simulink model "FullModelSimulation"  (R2021b)
settings: Solver=VariableStepAuto  StartTime=0.0  StopTime=24*3600  RelTol=1e-3
values from neighbouring files (symbols this model uses):
  A = double(A)    [ComponentUnitTests.m]    (also in ComponentUnitTests_linerization.m; InnerLoopNonLinSim.m; Kalman_filter_v2.m = [-0.3236   -0.0406   -0.1577   10.0671   -0.7623    0.0000)
  K = 5.4274    [Kalman_filter_final.m]
  ts = 0.025    [ComponentUnitTests.m]    (also in ComponentUnitTests_linerization.m; InnerLoopNonLinSim.m; Kalman_filter_final.m = 1; Kalman_filter_v2.m)
undefined symbols (not defined in the file or in its folder): Bp, Discrete, Time
libraries: slpidlib x2, ctrlSharedLib x1, TankPressure_Lib x1, VelocityDALQR_lib x1
settings Model: Creator=Christian  LastModifiedBy=Christian
settings SolverCC: AlgebraicLoopSolver=TrustRegion
settings DebuggingCC: SFMachineParentedDataDiag=warning

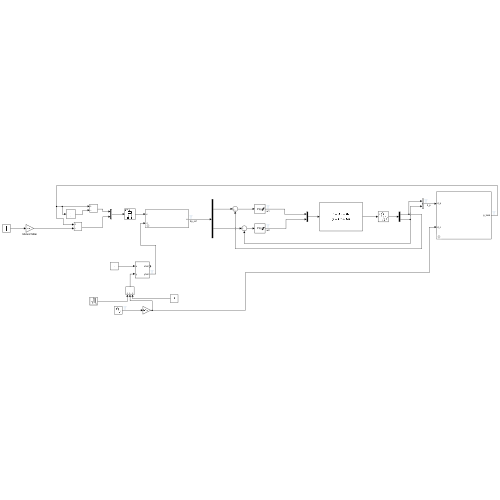
[thumbnail: Simulink's stored preview of the top-level diagram]
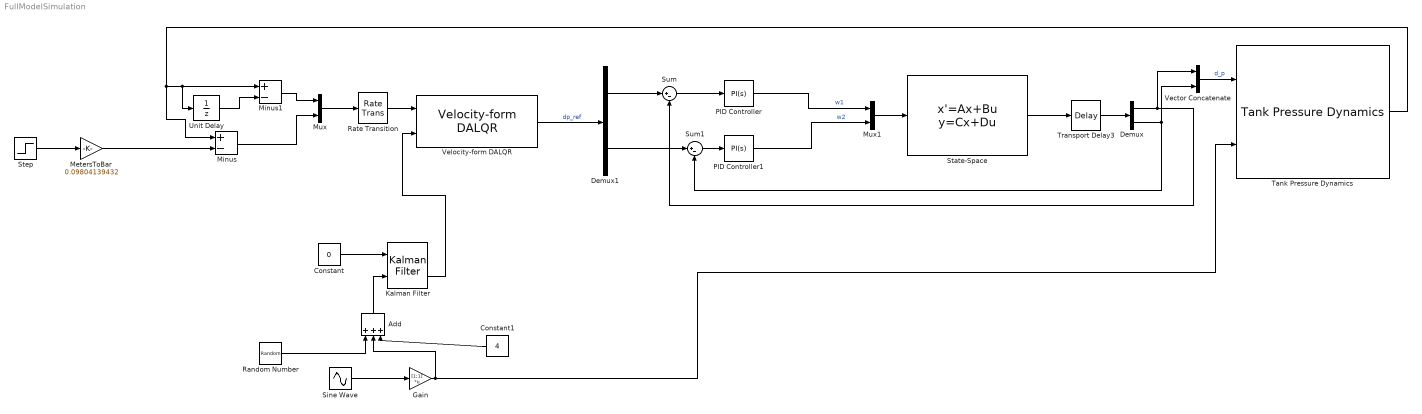
== system FullModelSimulation ==
  Add : Sum  Inputs=+++
  Constant : Constant  Value=0
  Constant1 : Constant  Value=4
  Demux : Demux  Outputs=2
  Demux1 : Demux  Outputs=2
  Gain : Gain  Gain=[1;1]  Multiplication=Matrix(K*u)
  Kalman Filter : ctrlSharedLib/Kalman Filter  TimeDomain=Discrete-Time  UseCurrentEstimator=on  ModelSource=LTI State-Space Variable  ModelSourceVariable=KalmSys  A=0.95  B=1  C=1  D=0  NumberOfStates=1  NumberOfInputs=1  NumberOfOutputs=1  InitialEstimateSource=Dialog  X0=0  P0=10  UseK=off  UseGH=off  NumberOfProcessNoiseInputs=1  G=1  TimeInvariantG=on  H=0  TimeInvariantH=on  Q=0.05  TimeInvariantQ=on  R=100  TimeInvariantR=on  N=0  TimeInvariantN=on  AddInputPort=on  AddEnablePort=off  OutputEstimatedY=on  OutputP=off  Ts=-1
  MetersToBar : Gain  Gain=0.09804139432
  Minus : Sum  Inputs=+-
  Minus1 : Sum  Inputs=+-
  Mux : Mux  Inputs=2
  Mux1 : Mux  Inputs=2
  PID Controller : slpidlib/PID Controller  Controller=PI  Form=Ideal  TimeDomain=Continuous-time  UseExternalTs=off  SampleTime=-1  IntegratorMethod=Forward Euler  FilterMethod=Forward Euler  ControllerParametersSource=internal  P=1.8  I=0.125  D=0  UseFilter=on  N=100  TunerSelectOption=Transfer Function Based (PID Tuner App)  InitialConditionSource=internal  InitialConditionForIntegrator=0  InitialConditionForFilter=0  DifferentiatorICPrevScaledInput=0  ExternalReset=none  TrackingMode=off  Kt=1  LimitOutput=on  SatLimitsSource=internal  UpperSaturationLimit=100  LowerSaturationLimit=0  LinearizeAsGain=on  AntiWindupMode=back-calculation  Kb=1  POutMin=[]  POutMax=[]  IOutMin=[]  IOutMax=[]  DOutMin=[]  DOutMax=[]  NOutMin=[]  NOutMax=[]  SumOutMin=[]  SumOutMax=[]  SaturationOutMin=[]  SaturationOutMax=[]  PParamMin=[]  PParamMax=[]  IParamMin=[]  IParamMax=[]  DParamMin=[]  DParamMax=[]  NParamMin=[]  NParamMax=[]  KbParamMin=[]  KbParamMax=[]  KtParamMin=[]  KtParamMax=[]  KbOutMin=[]  KbOutMax=[]  KtOutMin=[]  KtOutMax=[]  IntegratorOutMin=[]  IntegratorOutMax=[]  FilterOutMin=[]  FilterOutMax=[]  SumI1OutMin=[]  SumI1OutMax=[]  SumI2OutMin=[]  SumI2OutMax=[]  SumI3OutMin=[]  SumI3OutMax=[]  SumI4OutMin=[]  SumI4OutMax=[]  SumDOutMin=[]  SumDOutMax=[]  DifferentiatorOutMin=[]  DifferentiatorOutMax=[]  FilterDiffOutCoefMin=[]  FilterDiffOutCoefMax=[]  ReciprocalOutMin=[]  ReciprocalOutMax=[]  SumDenOutMin=[]  SumDenOutMax=[]  SumNumOutMin=[]  SumNumOutMax=[]  DivideOutMin=[]  DivideOutMax=[]  UdiffTsProdOutMin=[]  UdiffTsProdOutMax=[]  NTsProdOutMin=[]  NTsProdOutMax=[]  UintegralTsProdOutMin=[]  UintegralTsProdOutMax=[]  UngainTsProdOutMin=[]  UngainTsProdOutMax=[]  IntegratorContinuousStateAttributes=''  IntegratorStateMustResolveToSignalObject=off  IntegratorRTWStateStorageClass=Auto  FilterContinuousStateAttributes=''  FilterStateMustResolveToSignalObject=off  FilterRTWStateStorageClass=Auto  ParallelPVariant=Passthrough  IdealPVariant=InternalParameters  IVariant=InternalParameters  DVariant=Disabled  IntegratorVariant=Continuous  SatVariant=Enabled  AWVariant=BackCalculation  PCopyVariant=Disabled  TRVariant=Disabled  FdbkBlocksVariant=Forward  IdealPFdbkVariant=Disabled  SatFdbkVariant=Disabled  DerivativeFilterVariant=Disabled  NVariant=Disabled  NCopyVariant=Disabled_SignalSpec  FilterICVariant=Disabled  IntegratorICVariant=InternalICs  ExternalResetVariant=Disabled  TRSumVariant=Passthrough  SumFdbkVariant=Disabled  SumVariant=Sum_PI  TsampFilterVariant=InternalTs  TsampNgainVariant=Passthrough  TsampIntegralVariant=Passthrough  ExternalSaturationOutDataTypeStr=Inherit: Same as second input
  PID Controller1 : slpidlib/PID Controller  Controller=PI  Form=Ideal  TimeDomain=Continuous-time  UseExternalTs=off  SampleTime=-1  IntegratorMethod=Forward Euler  FilterMethod=Forward Euler  ControllerParametersSource=internal  P=1.8  I=0.125  D=0  UseFilter=on  N=100  TunerSelectOption=Transfer Function Based (PID Tuner App)  InitialConditionSource=internal  InitialConditionForIntegrator=0  InitialConditionForFilter=0  DifferentiatorICPrevScaledInput=0  ExternalReset=none  TrackingMode=off  Kt=1  LimitOutput=on  SatLimitsSource=internal  UpperSaturationLimit=100  LowerSaturationLimit=0  LinearizeAsGain=on  AntiWindupMode=back-calculation  Kb=1  POutMin=[]  POutMax=[]  IOutMin=[]  IOutMax=[]  DOutMin=[]  DOutMax=[]  NOutMin=[]  NOutMax=[]  SumOutMin=[]  SumOutMax=[]  SaturationOutMin=[]  SaturationOutMax=[]  PParamMin=[]  PParamMax=[]  IParamMin=[]  IParamMax=[]  DParamMin=[]  DParamMax=[]  NParamMin=[]  NParamMax=[]  KbParamMin=[]  KbParamMax=[]  KtParamMin=[]  KtParamMax=[]  KbOutMin=[]  KbOutMax=[]  KtOutMin=[]  KtOutMax=[]  IntegratorOutMin=[]  IntegratorOutMax=[]  FilterOutMin=[]  FilterOutMax=[]  SumI1OutMin=[]  SumI1OutMax=[]  SumI2OutMin=[]  SumI2OutMax=[]  SumI3OutMin=[]  SumI3OutMax=[]  SumI4OutMin=[]  SumI4OutMax=[]  SumDOutMin=[]  SumDOutMax=[]  DifferentiatorOutMin=[]  DifferentiatorOutMax=[]  FilterDiffOutCoefMin=[]  FilterDiffOutCoefMax=[]  ReciprocalOutMin=[]  ReciprocalOutMax=[]  SumDenOutMin=[]  SumDenOutMax=[]  SumNumOutMin=[]  SumNumOutMax=[]  DivideOutMin=[]  DivideOutMax=[]  UdiffTsProdOutMin=[]  UdiffTsProdOutMax=[]  NTsProdOutMin=[]  NTsProdOutMax=[]  UintegralTsProdOutMin=[]  UintegralTsProdOutMax=[]  UngainTsProdOutMin=[]  UngainTsProdOutMax=[]  IntegratorContinuousStateAttributes=''  IntegratorStateMustResolveToSignalObject=off  IntegratorRTWStateStorageClass=Auto  FilterContinuousStateAttributes=''  FilterStateMustResolveToSignalObject=off  FilterRTWStateStorageClass=Auto  ParallelPVariant=Passthrough  IdealPVariant=InternalParameters  IVariant=InternalParameters  DVariant=Disabled  IntegratorVariant=Continuous  SatVariant=Enabled  AWVariant=BackCalculation  PCopyVariant=Disabled  TRVariant=Disabled  FdbkBlocksVariant=Forward  IdealPFdbkVariant=Disabled  SatFdbkVariant=Disabled  DerivativeFilterVariant=Disabled  NVariant=Disabled  NCopyVariant=Disabled_SignalSpec  FilterICVariant=Disabled  IntegratorICVariant=InternalICs  ExternalResetVariant=Disabled  TRSumVariant=Passthrough  SumFdbkVariant=Disabled  SumVariant=Sum_PI  TsampFilterVariant=InternalTs  TsampNgainVariant=Passthrough  TsampIntegralVariant=Passthrough  ExternalSaturationOutDataTypeStr=Inherit: Same as second input
  Random Number : RandomNumber  Mean=[0;0]  Variance=[0.1;0.1]  SampleTime=10  VectorParams1D=off
  Rate Transition : RateTransition  OutPortSampleTime=100
  Sine Wave : Sin  Amplitude=2  Bias=-2  Frequency=2*pi*1/(12*3600)  SampleTime=10
  State-Space : StateSpace  A=|  B=|  C=|  D=[0 0 ; 0 0]  InitialCondition=0
      A=|
      | [-0.3236   -0.0406   -0.1577   10.0671   -0.7623    0.0000;
      |    -0.1429   -0.3189    0.2176   -1.3489   -6.0984         0;
      |    -0.0275    0.0687   -0.3968    7.1758    1.5246         0;
      |     0.1089    0.0687    0.0196  -20.2792    1.5246   -0.0000;
      |    -0.0551   -0.0443   -0.0272    1.4425  -15.3466   -0.0999;
      |     0.1486    0.0817   -0.2877   11.1436    8.2419   -0.4174]
      B=|
      | [0.0982    0.0000;
      |     0.0078         0;
      |     0.1147         0;
      |    -0.0408         0;
      |    -0.0087   -0.0193;
      |    -0.0651   -0.0715]
      C=|
      | [0 0 1 0 0 0;
      | 	0 0 -1 -1 -1 -1]
  Step : Step  Time=12*3600  Before=2  After=5  SampleTime=0
  Sum : Sum  Inputs=|+-
  Sum1 : Sum  Inputs=|+-
  Tank Pressure Dynamics : TankPressure_Lib/Tank Pressure Dynamics  p_0=1*0.09804139432  A=A  B_producer=Bp  B_consumer=Bc  Ts=ts
  Transport Delay3 : TransportDelay  DelayTime=4  InitialOutput=[0;0]
  Unit Delay : UnitDelay  InitialCondition=1  SampleTime=-1  HasFrameUpgradeWarning=on
  Vector Concatenate : Concatenate
  Velocity-form DALQR : VelocityDALQR_lib/Velocity-form DALQR  K=K  B_disturbance=Bc  B=Bp
  wires:
  Mux/1 -> Rate Transition/1
  Unit Delay/1 -> Minus1/2
  Tank Pressure Dynamics/1 -> Minus/1, Unit Delay/1, Minus1/1
  Minus/1 -> Mux/2
  Step/1 -> MetersToBar/1
  Minus1/1 -> Mux/1
  Sum/1 -> PID Controller/1
  PID Controller/1 -> Mux1/1  "w1"
  Sum1/1 -> PID Controller1/1
  Demux/2 -> Vector Concatenate/2, Sum1/2
  Demux/1 -> Vector Concatenate/1, Sum/2
  PID Controller1/1 -> Mux1/2  "w2"
  Transport Delay3/1 -> Demux/1
  State-Space/1 -> Transport Delay3/1
  Mux1/1 -> State-Space/1
  Velocity-form DALQR/1 -> Demux1/1  "dp_ref"
  Demux1/1 -> Sum/1
  Demux1/2 -> Sum1/1
  Rate Transition/1 -> Velocity-form DALQR/1
  Vector Concatenate/1 -> Tank Pressure Dynamics/1  "d_p"
  Sine Wave/1 -> Gain/1
  Gain/1 -> Add/2, Tank Pressure Dynamics/2
  Constant/1 -> Kalman Filter/1
  Random Number/1 -> Add/1
  Add/1 -> Kalman Filter/2
  Kalman Filter/2 -> Velocity-form DALQR/2
  Constant1/1 -> Add/3
  MetersToBar/1 -> Minus/2
